simulink model "gm_uz_pmsm_model_9ph"  (R2021b)
settings: Solver=FixedStepAuto  StartTime=0.0  StopTime=0.8  RelTol=1e-3
PreLoadFcn:
  | uz_pmsm_model_9ph_init_parameter
undefined symbols (not defined in the file or in its folder): a, b, c, friction_coefficient, inertia, k_i_d, k_i_q, k_p_d, k_p_q, Kpd, L_d, L_o1, L_o2, L_q, L_x1, L_x2, L_y1, L_y2, L_zero, polepair, psi_pm, R_1, static_friction_torque, Tnd
libraries: hdlmdlgenlib x190, hdlsllib x90, dspsigops x17, simulink x3, slpidlib x2, spsAlphaBetaZerotodq0Lib x1, pid_lib x1, spsdq0toAlphaBetaZeroLib x1
(part 3 of 6)

== system gm_uz_pmsm_model_9ph/Subsystem8/Subsystem3 ==
  setp_Mod_x : Inport
  actual_Mod_x : Inport  Port=2
  Add : Sum  Inputs=+-
  Data Type Conversion8 : DataTypeConversion  OutDataTypeStr=double
  PID Controller2 : slpidlib/PID Controller  Controller=PI  Form=Ideal  TimeDomain=Continuous-time  UseExternalTs=off  SampleTime=-1  IntegratorMethod=Forward Euler  FilterMethod=Forward Euler  ControllerParametersSource=internal  P=k_p_q  I=k_i_q  D=0  UseFilter=on  N=100  TunerSelectOption=Transfer Function Based (PID Tuner App)  InitialConditionSource=internal  InitialConditionForIntegrator=0  InitialConditionForFilter=0  DifferentiatorICPrevScaledInput=0  ExternalReset=none  TrackingMode=off  Kt=1  LimitOutput=on  SatLimitsSource=internal  UpperSaturationLimit=100  LowerSaturationLimit=-100  LinearizeAsGain=on  AntiWindupMode=clamping  Kb=1  POutMin=[]  POutMax=[]  IOutMin=[]  IOutMax=[]  DOutMin=[]  DOutMax=[]  NOutMin=[]  NOutMax=[]  SumOutMin=[]  SumOutMax=[]  SaturationOutMin=[]  SaturationOutMax=[]  PParamMin=[]  PParamMax=[]  IParamMin=[]  IParamMax=[]  DParamMin=[]  DParamMax=[]  NParamMin=[]  NParamMax=[]  KbParamMin=[]  KbParamMax=[]  KtParamMin=[]  KtParamMax=[]  KbOutMin=[]  KbOutMax=[]  KtOutMin=[]  KtOutMax=[]  IntegratorOutMin=[]  IntegratorOutMax=[]  FilterOutMin=[]  FilterOutMax=[]  SumI1OutMin=[]  SumI1OutMax=[]  SumI2OutMin=[]  SumI2OutMax=[]  SumI3OutMin=[]  SumI3OutMax=[]  SumI4OutMin=[]  SumI4OutMax=[]  SumDOutMin=[]  SumDOutMax=[]  DifferentiatorOutMin=[]  DifferentiatorOutMax=[]  FilterDiffOutCoefMin=[]  FilterDiffOutCoefMax=[]  ReciprocalOutMin=[]  ReciprocalOutMax=[]  SumDenOutMin=[]  SumDenOutMax=[]  SumNumOutMin=[]  SumNumOutMax=[]  DivideOutMin=[]  DivideOutMax=[]  UdiffTsProdOutMin=[]  UdiffTsProdOutMax=[]  NTsProdOutMin=[]  NTsProdOutMax=[]  UintegralTsProdOutMin=[]  UintegralTsProdOutMax=[]  UngainTsProdOutMin=[]  UngainTsProdOutMax=[]  IntegratorContinuousStateAttributes=''  IntegratorStateMustResolveToSignalObject=off  IntegratorRTWStateStorageClass=Auto  FilterContinuousStateAttributes=''  FilterStateMustResolveToSignalObject=off  FilterRTWStateStorageClass=Auto  ParallelPVariant=Passthrough  IdealPVariant=InternalParameters  IVariant=InternalParameters  DVariant=Disabled  IntegratorVariant=Continuous  SatVariant=Enabled  AWVariant=ContClampingIdeal  PCopyVariant=InternalParamsIdeal  TRVariant=Disabled  FdbkBlocksVariant=Forward  IdealPFdbkVariant=Disabled  SatFdbkVariant=Disabled  DerivativeFilterVariant=Disabled  NVariant=Disabled  NCopyVariant=Disabled_SignalSpec  FilterICVariant=Disabled  IntegratorICVariant=InternalICs  ExternalResetVariant=Disabled  TRSumVariant=Passthrough  SumFdbkVariant=Disabled  SumVariant=Sum_PI  TsampFilterVariant=InternalTs  TsampNgainVariant=Passthrough  TsampIntegralVariant=Passthrough  ExternalSaturationOutDataTypeStr=Inherit: Same as second input
  out_mod_x : Outport
  wires:
  Add/1 -> Data Type Conversion8/1
  actual_Mod_x/1 -> Add/2
  Data Type Conversion8/1 -> PID Controller2/1
  setp_Mod_x/1 -> Add/1
  PID Controller2/1 -> out_mod_x/1

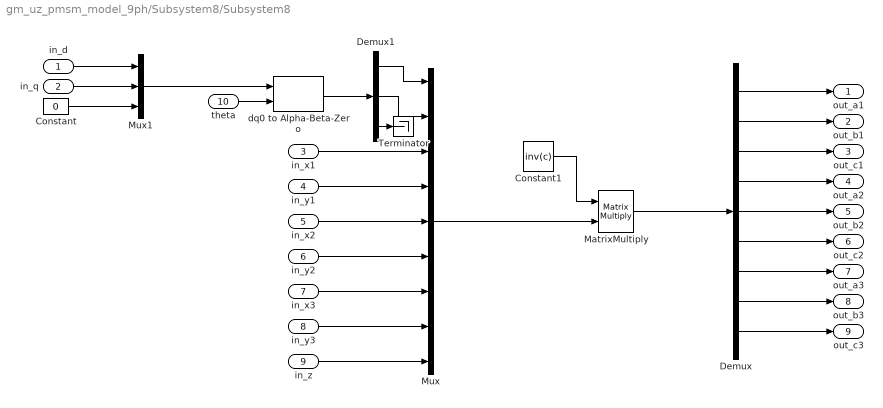
== system gm_uz_pmsm_model_9ph/Subsystem8/Subsystem8 ==
  in_d : Inport
  in_q : Inport  Port=2
  in_x1 : Inport  Port=3
  in_y1 : Inport  Port=4
  in_x2 : Inport  Port=5
  in_y2 : Inport  Port=6
  in_x3 : Inport  Port=7
  in_y3 : Inport  Port=8
  in_z : Inport  Port=9
  theta : Inport  Port=10
  Constant : Constant  Value=0
  Constant1 : Constant  Value=inv(c)
  Demux : Demux  Outputs=9
  Demux1 : Demux  Outputs=3
  MatrixMultiply : Product  Multiplication=Matrix(*)
  Mux : Mux  Inputs=9
  Mux1 : Mux  Inputs=3
  Terminator : Terminator
  dq0 to Alpha-Beta-Zero : spsdq0toAlphaBetaZeroLib/dq0 to Alpha-Beta-Zero  Alignment=90 degrees behind phase A axis
      settings: SourceProductBaseCode=PS
  out_a1 : Outport
  out_b1 : Outport  Port=2
  out_c1 : Outport  Port=3
  out_a2 : Outport  Port=4
  out_b2 : Outport  Port=5
  out_c2 : Outport  Port=6
  out_a3 : Outport  Port=7
  out_b3 : Outport  Port=8
  out_c3 : Outport  Port=9
  wires:
  Demux/7 -> out_a3/1
  Demux/9 -> out_c3/1
  Demux/8 -> out_b3/1
  Demux/5 -> out_b2/1
  Demux/6 -> out_c2/1
  Demux/4 -> out_a2/1
  Demux/3 -> out_c1/1
  Demux/2 -> out_b1/1
  Constant1/1 -> MatrixMultiply/1
  Demux1/3 -> Terminator/1
  Demux1/2 -> Mux/2
  Demux1/1 -> Mux/1
  dq0 to Alpha-Beta-Zero/1 -> Demux1/1
  theta/1 -> dq0 to Alpha-Beta-Zero/2
  Mux1/1 -> dq0 to Alpha-Beta-Zero/1
  in_d/1 -> Mux1/1
  in_q/1 -> Mux1/2
  Constant/1 -> Mux1/3
  in_z/1 -> Mux/9
  in_x2/1 -> Mux/5
  Mux/1 -> MatrixMultiply/2
  in_y1/1 -> Mux/4
  in_x1/1 -> Mux/3
  Demux/1 -> out_a1/1
  in_y2/1 -> Mux/6
  MatrixMultiply/1 -> Demux/1
  in_y3/1 -> Mux/8
  in_x3/1 -> Mux/7

== system gm_uz_pmsm_model_9ph/uz_pmsm_model_9ph/Add ==
  In1 : Inport
  In2 : Inport  Port=2
  Add : Sum  Inputs=+-  OutDataTypeStr=single  SampleTime=1e-08
  Add_pd1 : Delay  DelayLength=6
  Out1 : Outport
  wires:
  In1/1 -> Add/1
  In2/1 -> Add/2
  Add/1 -> Add_pd1/1
  Add_pd1/1 -> Out1/1

== system gm_uz_pmsm_model_9ph/uz_pmsm_model_9ph/Add1 ==
  In1 : Inport
  In2 : Inport  Port=2
  Add1 : Sum  Inputs=+-  OutDataTypeStr=single  SampleTime=1e-08
  Add1_pd1 : Delay  DelayLength=6
  Out1 : Outport
  wires:
  In1/1 -> Add1/1
  In2/1 -> Add1/2
  Add1/1 -> Add1_pd1/1
  Add1_pd1/1 -> Out1/1

== system gm_uz_pmsm_model_9ph/uz_pmsm_model_9ph/Add2 ==
  In1 : Inport
  In2 : Inport  Port=2
  Add2 : Sum  Inputs=+-  OutDataTypeStr=single  SampleTime=1e-08
  Add2_pd1 : Delay  DelayLength=6
  Out1 : Outport
  wires:
  In1/1 -> Add2/1
  In2/1 -> Add2/2
  Add2/1 -> Add2_pd1/1
  Add2_pd1/1 -> Out1/1

== system gm_uz_pmsm_model_9ph/uz_pmsm_model_9ph/Add3 ==
  In1 : Inport
  In2 : Inport  Port=2
  Add3 : Sum  Inputs=+-  OutDataTypeStr=single  SampleTime=1e-08
  Add3_pd1 : Delay  DelayLength=6
  Out1 : Outport
  wires:
  In1/1 -> Add3/1
  In2/1 -> Add3/2
  Add3/1 -> Add3_pd1/1
  Add3_pd1/1 -> Out1/1

== system gm_uz_pmsm_model_9ph/uz_pmsm_model_9ph/Add4 ==
  In1 : Inport
  In2 : Inport  Port=2
  Add4 : Sum  Inputs=+-  OutDataTypeStr=single  SampleTime=1e-08
  Add4_pd1 : Delay  DelayLength=6
  Out1 : Outport
  wires:
  In1/1 -> Add4/1
  In2/1 -> Add4/2
  Add4/1 -> Add4_pd1/1
  Add4_pd1/1 -> Out1/1

== system gm_uz_pmsm_model_9ph/uz_pmsm_model_9ph/Add5 ==
  In1 : Inport
  In2 : Inport  Port=2
  Add5 : Sum  Inputs=+-  OutDataTypeStr=single  SampleTime=1e-08
  Add5_pd1 : Delay  DelayLength=6
  Out1 : Outport
  wires:
  In1/1 -> Add5/1
  In2/1 -> Add5/2
  Add5/1 -> Add5_pd1/1
  Add5_pd1/1 -> Out1/1

== system gm_uz_pmsm_model_9ph/uz_pmsm_model_9ph/Add6 ==
  In1 : Inport
  In2 : Inport  Port=2
  Add6 : Sum  Inputs=+-  OutDataTypeStr=single  SampleTime=1e-08
  Add6_pd1 : Delay  DelayLength=6
  Out1 : Outport
  wires:
  In1/1 -> Add6/1
  In2/1 -> Add6/2
  Add6/1 -> Add6_pd1/1
  Add6_pd1/1 -> Out1/1

== system gm_uz_pmsm_model_9ph/uz_pmsm_model_9ph/Cast To Double ==
  In1 : Inport
  Cast To Double : DataTypeConversion  OutDataTypeStr=single  SampleTime=1e-08
  Cast To Double_pd1 : Delay  DelayLength=6
  Out1 : Outport
  wires:
  In1/1 -> Cast To Double/1
  Cast To Double/1 -> Cast To Double_pd1/1
  Cast To Double_pd1/1 -> Out1/1

== system gm_uz_pmsm_model_9ph/uz_pmsm_model_9ph/Cast To Double1 ==
  In1 : Inport
  Cast To Double1 : DataTypeConversion  OutDataTypeStr=single  SampleTime=1e-08
  Cast To Double1_pd1 : Delay  DelayLength=6
  Out1 : Outport
  wires:
  In1/1 -> Cast To Double1/1
  Cast To Double1/1 -> Cast To Double1_pd1/1
  Cast To Double1_pd1/1 -> Out1/1

== system gm_uz_pmsm_model_9ph/uz_pmsm_model_9ph/Cast To Double2 ==
  In1 : Inport
  Cast To Double2 : DataTypeConversion  OutDataTypeStr=single  SampleTime=1e-08
  Cast To Double2_pd1 : Delay  DelayLength=6
  Out1 : Outport
  wires:
  In1/1 -> Cast To Double2/1
  Cast To Double2/1 -> Cast To Double2_pd1/1
  Cast To Double2_pd1/1 -> Out1/1

== system gm_uz_pmsm_model_9ph/uz_pmsm_model_9ph/Data Type Conversion1 ==
  In1 : Inport
  Data Type Conversion1 : DataTypeConversion  OutDataTypeStr=fixdt(1, 25, 12)  RndMeth=Nearest  SampleTime=1e-08
  Data Type Conversion1_pd1 : Delay  DelayLength=6
  Out1 : Outport
  wires:
  In1/1 -> Data Type Conversion1/1
  Data Type Conversion1/1 -> Data Type Conversion1_pd1/1
  Data Type Conversion1_pd1/1 -> Out1/1

== system gm_uz_pmsm_model_9ph/uz_pmsm_model_9ph/Data Type Conversion11 ==
  In1 : Inport
  Data Type Conversion11 : DataTypeConversion  OutDataTypeStr=double  RndMeth=Nearest  SampleTime=1e-08
  Data Type Conversion11_pd1 : Delay  DelayLength=3
  Out1 : Outport
  wires:
  In1/1 -> Data Type Conversion11/1
  Data Type Conversion11/1 -> Data Type Conversion11_pd1/1
  Data Type Conversion11_pd1/1 -> Out1/1

== system gm_uz_pmsm_model_9ph/uz_pmsm_model_9ph/Data Type Conversion12 ==
  In1 : Inport
  Data Type Conversion12 : DataTypeConversion  OutDataTypeStr=double  RndMeth=Nearest  SampleTime=1e-08
  Data Type Conversion12_pd1 : Delay  DelayLength=3
  Out1 : Outport
  wires:
  In1/1 -> Data Type Conversion12/1
  Data Type Conversion12/1 -> Data Type Conversion12_pd1/1
  Data Type Conversion12_pd1/1 -> Out1/1

== system gm_uz_pmsm_model_9ph/uz_pmsm_model_9ph/Data Type Conversion13 ==
  In1 : Inport
  Data Type Conversion13 : DataTypeConversion  OutDataTypeStr=single  RndMeth=Nearest  SampleTime=1e-08
  Data Type Conversion13_pd1 : Delay  DelayLength=3
  Out1 : Outport
  wires:
  In1/1 -> Data Type Conversion13/1
  Data Type Conversion13/1 -> Data Type Conversion13_pd1/1
  Data Type Conversion13_pd1/1 -> Out1/1

== system gm_uz_pmsm_model_9ph/uz_pmsm_model_9ph/Data Type Conversion14 ==
  In1 : Inport
  Data Type Conversion14 : DataTypeConversion  OutDataTypeStr=double  RndMeth=Nearest  SampleTime=1e-08
  Data Type Conversion14_pd1 : Delay  DelayLength=3
  Out1 : Outport
  wires:
  In1/1 -> Data Type Conversion14/1
  Data Type Conversion14/1 -> Data Type Conversion14_pd1/1
  Data Type Conversion14_pd1/1 -> Out1/1

== system gm_uz_pmsm_model_9ph/uz_pmsm_model_9ph/Data Type Conversion141 ==
  In1 : Inport
  Data Type Conversion141 : DataTypeConversion  OutDataTypeStr=single  RndMeth=Nearest  SampleTime=1e-08
  Data Type Conversion141_pd1 : Delay  DelayLength=3
  Out1 : Outport
  wires:
  In1/1 -> Data Type Conversion141/1
  Data Type Conversion141/1 -> Data Type Conversion141_pd1/1
  Data Type Conversion141_pd1/1 -> Out1/1

== system gm_uz_pmsm_model_9ph/uz_pmsm_model_9ph/Data Type Conversion15 ==
  In1 : Inport
  Data Type Conversion15 : DataTypeConversion  OutDataTypeStr=single  RndMeth=Nearest  SampleTime=1e-08
  Data Type Conversion15_pd1 : Delay  DelayLength=3
  Out1 : Outport
  wires:
  In1/1 -> Data Type Conversion15/1
  Data Type Conversion15/1 -> Data Type Conversion15_pd1/1
  Data Type Conversion15_pd1/1 -> Out1/1

== system gm_uz_pmsm_model_9ph/uz_pmsm_model_9ph/Data Type Conversion16 ==
  In1 : Inport
  Data Type Conversion16 : DataTypeConversion  OutDataTypeStr=single  RndMeth=Nearest  SampleTime=1e-08
  Data Type Conversion16_pd1 : Delay  DelayLength=3
  Out1 : Outport
  wires:
  In1/1 -> Data Type Conversion16/1
  Data Type Conversion16/1 -> Data Type Conversion16_pd1/1
  Data Type Conversion16_pd1/1 -> Out1/1

== system gm_uz_pmsm_model_9ph/uz_pmsm_model_9ph/Data Type Conversion17 ==
  In1 : Inport
  Data Type Conversion17 : DataTypeConversion  OutDataTypeStr=single  RndMeth=Nearest  SampleTime=1e-08
  Data Type Conversion17_pd1 : Delay  DelayLength=3
  Out1 : Outport
  wires:
  In1/1 -> Data Type Conversion17/1
  Data Type Conversion17/1 -> Data Type Conversion17_pd1/1
  Data Type Conversion17_pd1/1 -> Out1/1

== system gm_uz_pmsm_model_9ph/uz_pmsm_model_9ph/Data Type Conversion18 ==
  In1 : Inport
  Data Type Conversion18 : DataTypeConversion  OutDataTypeStr=single  RndMeth=Nearest  SampleTime=1e-08
  Data Type Conversion18_pd1 : Delay  DelayLength=3
  Out1 : Outport
  wires:
  In1/1 -> Data Type Conversion18/1
  Data Type Conversion18/1 -> Data Type Conversion18_pd1/1
  Data Type Conversion18_pd1/1 -> Out1/1

== system gm_uz_pmsm_model_9ph/uz_pmsm_model_9ph/Data Type Conversion19 ==
  In1 : Inport
  Data Type Conversion19 : DataTypeConversion  OutDataTypeStr=single  RndMeth=Nearest  SampleTime=1e-08
  Data Type Conversion19_pd1 : Delay  DelayLength=3
  Out1 : Outport
  wires:
  In1/1 -> Data Type Conversion19/1
  Data Type Conversion19/1 -> Data Type Conversion19_pd1/1
  Data Type Conversion19_pd1/1 -> Out1/1

== system gm_uz_pmsm_model_9ph/uz_pmsm_model_9ph/Data Type Conversion20 ==
  In1 : Inport
  Data Type Conversion20 : DataTypeConversion  OutDataTypeStr=single  RndMeth=Nearest  SampleTime=1e-08
  Data Type Conversion20_pd1 : Delay  DelayLength=3
  Out1 : Outport
  wires:
  In1/1 -> Data Type Conversion20/1
  Data Type Conversion20/1 -> Data Type Conversion20_pd1/1
  Data Type Conversion20_pd1/1 -> Out1/1

== system gm_uz_pmsm_model_9ph/uz_pmsm_model_9ph/Data Type Conversion21 ==
  In1 : Inport
  Data Type Conversion21 : DataTypeConversion  OutDataTypeStr=double  RndMeth=Nearest  SampleTime=1e-08
  Data Type Conversion21_pd1 : Delay  DelayLength=3
  Out1 : Outport
  wires:
  In1/1 -> Data Type Conversion21/1
  Data Type Conversion21/1 -> Data Type Conversion21_pd1/1
  Data Type Conversion21_pd1/1 -> Out1/1

== system gm_uz_pmsm_model_9ph/uz_pmsm_model_9ph/Data Type Conversion22 ==
  In1 : Inport
  Data Type Conversion22 : DataTypeConversion  OutDataTypeStr=double  RndMeth=Nearest  SampleTime=1e-08
  Data Type Conversion22_pd1 : Delay  DelayLength=3
  Out1 : Outport
  wires:
  In1/1 -> Data Type Conversion22/1
  Data Type Conversion22/1 -> Data Type Conversion22_pd1/1
  Data Type Conversion22_pd1/1 -> Out1/1

== system gm_uz_pmsm_model_9ph/uz_pmsm_model_9ph/Data Type Conversion23 ==
  In1 : Inport
  Data Type Conversion23 : DataTypeConversion  OutDataTypeStr=single  RndMeth=Nearest  SampleTime=1e-08
  Data Type Conversion23_pd1 : Delay  DelayLength=3
  Out1 : Outport
  wires:
  In1/1 -> Data Type Conversion23/1
  Data Type Conversion23/1 -> Data Type Conversion23_pd1/1
  Data Type Conversion23_pd1/1 -> Out1/1

== system gm_uz_pmsm_model_9ph/uz_pmsm_model_9ph/Data Type Conversion24 ==
  In1 : Inport
  Data Type Conversion24 : DataTypeConversion  OutDataTypeStr=double  RndMeth=Nearest  SampleTime=1e-08
  Data Type Conversion24_pd1 : Delay  DelayLength=3
  Out1 : Outport
  wires:
  In1/1 -> Data Type Conversion24/1
  Data Type Conversion24/1 -> Data Type Conversion24_pd1/1
  Data Type Conversion24_pd1/1 -> Out1/1

== system gm_uz_pmsm_model_9ph/uz_pmsm_model_9ph/Data Type Conversion25 ==
  In1 : Inport
  Data Type Conversion25 : DataTypeConversion  OutDataTypeStr=double  RndMeth=Nearest  SampleTime=1e-08
  Data Type Conversion25_pd1 : Delay  DelayLength=3
  Out1 : Outport
  wires:
  In1/1 -> Data Type Conversion25/1
  Data Type Conversion25/1 -> Data Type Conversion25_pd1/1
  Data Type Conversion25_pd1/1 -> Out1/1

== system gm_uz_pmsm_model_9ph/uz_pmsm_model_9ph/Data Type Conversion26 ==
  In1 : Inport
  Data Type Conversion26 : DataTypeConversion  OutDataTypeStr=double  RndMeth=Nearest  SampleTime=1e-08
  Data Type Conversion26_pd1 : Delay  DelayLength=3
  Out1 : Outport
  wires:
  In1/1 -> Data Type Conversion26/1
  Data Type Conversion26/1 -> Data Type Conversion26_pd1/1
  Data Type Conversion26_pd1/1 -> Out1/1

== system gm_uz_pmsm_model_9ph/uz_pmsm_model_9ph/Data Type Conversion27 ==
  In1 : Inport
  Data Type Conversion27 : DataTypeConversion  OutDataTypeStr=double  RndMeth=Nearest  SampleTime=1e-08
  Data Type Conversion27_pd1 : Delay  DelayLength=3
  Out1 : Outport
  wires:
  In1/1 -> Data Type Conversion27/1
  Data Type Conversion27/1 -> Data Type Conversion27_pd1/1
  Data Type Conversion27_pd1/1 -> Out1/1

== system gm_uz_pmsm_model_9ph/uz_pmsm_model_9ph/Data Type Conversion28 ==
  In1 : Inport
  Data Type Conversion28 : DataTypeConversion  OutDataTypeStr=double  RndMeth=Nearest  SampleTime=1e-08
  Data Type Conversion28_pd1 : Delay  DelayLength=3
  Out1 : Outport
  wires:
  In1/1 -> Data Type Conversion28/1
  Data Type Conversion28/1 -> Data Type Conversion28_pd1/1
  Data Type Conversion28_pd1/1 -> Out1/1

== system gm_uz_pmsm_model_9ph/uz_pmsm_model_9ph/Data Type Conversion29 ==
  In1 : Inport
  Data Type Conversion29 : DataTypeConversion  OutDataTypeStr=double  RndMeth=Nearest  SampleTime=1e-08
  Data Type Conversion29_pd1 : Delay  DelayLength=3
  Out1 : Outport
  wires:
  In1/1 -> Data Type Conversion29/1
  Data Type Conversion29/1 -> Data Type Conversion29_pd1/1
  Data Type Conversion29_pd1/1 -> Out1/1

== system gm_uz_pmsm_model_9ph/uz_pmsm_model_9ph/Data Type Conversion3 ==
  In1 : Inport
  Data Type Conversion3 : DataTypeConversion  OutDataTypeStr=double  RndMeth=Nearest  SampleTime=1e-08
  Data Type Conversion3_pd1 : Delay  DelayLength=3
  Out1 : Outport
  wires:
  In1/1 -> Data Type Conversion3/1
  Data Type Conversion3/1 -> Data Type Conversion3_pd1/1
  Data Type Conversion3_pd1/1 -> Out1/1

== system gm_uz_pmsm_model_9ph/uz_pmsm_model_9ph/Data Type Conversion30 ==
  In1 : Inport
  Data Type Conversion30 : DataTypeConversion  OutDataTypeStr=double  RndMeth=Nearest  SampleTime=1e-08
  Data Type Conversion30_pd1 : Delay  DelayLength=3
  Out1 : Outport
  wires:
  In1/1 -> Data Type Conversion30/1
  Data Type Conversion30/1 -> Data Type Conversion30_pd1/1
  Data Type Conversion30_pd1/1 -> Out1/1

== system gm_uz_pmsm_model_9ph/uz_pmsm_model_9ph/Data Type Conversion31 ==
  In1 : Inport
  Data Type Conversion31 : DataTypeConversion  OutDataTypeStr=single  RndMeth=Nearest  SampleTime=1e-08
  Data Type Conversion31_pd1 : Delay  DelayLength=3
  Out1 : Outport
  wires:
  In1/1 -> Data Type Conversion31/1
  Data Type Conversion31/1 -> Data Type Conversion31_pd1/1
  Data Type Conversion31_pd1/1 -> Out1/1

== system gm_uz_pmsm_model_9ph/uz_pmsm_model_9ph/Data Type Conversion32 ==
  In1 : Inport
  Data Type Conversion32 : DataTypeConversion  OutDataTypeStr=single  RndMeth=Nearest  SampleTime=1e-08
  Data Type Conversion32_pd1 : Delay  DelayLength=3
  Out1 : Outport
  wires:
  In1/1 -> Data Type Conversion32/1
  Data Type Conversion32/1 -> Data Type Conversion32_pd1/1
  Data Type Conversion32_pd1/1 -> Out1/1

== system gm_uz_pmsm_model_9ph/uz_pmsm_model_9ph/Data Type Conversion33 ==
  In1 : Inport
  Data Type Conversion33 : DataTypeConversion  OutDataTypeStr=double  RndMeth=Nearest  SampleTime=1e-08
  Data Type Conversion33_pd1 : Delay  DelayLength=3
  Out1 : Outport
  wires:
  In1/1 -> Data Type Conversion33/1
  Data Type Conversion33/1 -> Data Type Conversion33_pd1/1
  Data Type Conversion33_pd1/1 -> Out1/1

== system gm_uz_pmsm_model_9ph/uz_pmsm_model_9ph/Data Type Conversion331 ==
  In1 : Inport
  Data Type Conversion331 : DataTypeConversion  OutDataTypeStr=double  RndMeth=Nearest  SampleTime=1e-08
  Data Type Conversion331_pd1 : Delay  DelayLength=3
  Out1 : Outport
  wires:
  In1/1 -> Data Type Conversion331/1
  Data Type Conversion331/1 -> Data Type Conversion331_pd1/1
  Data Type Conversion331_pd1/1 -> Out1/1

== system gm_uz_pmsm_model_9ph/uz_pmsm_model_9ph/Data Type Conversion37 ==
  In1 : Inport
  Data Type Conversion37 : DataTypeConversion  OutDataTypeStr=single  RndMeth=Nearest  SampleTime=1e-08
  Data Type Conversion37_pd1 : Delay  DelayLength=6
  Out1 : Outport
  wires:
  In1/1 -> Data Type Conversion37/1
  Data Type Conversion37/1 -> Data Type Conversion37_pd1/1
  Data Type Conversion37_pd1/1 -> Out1/1

== system gm_uz_pmsm_model_9ph/uz_pmsm_model_9ph/Data Type Conversion5 ==
  In1 : Inport
  Data Type Conversion5 : DataTypeConversion  OutDataTypeStr=double  RndMeth=Nearest  SampleTime=1e-08
  Data Type Conversion5_pd1 : Delay  DelayLength=3
  Out1 : Outport
  wires:
  In1/1 -> Data Type Conversion5/1
  Data Type Conversion5/1 -> Data Type Conversion5_pd1/1
  Data Type Conversion5_pd1/1 -> Out1/1

== system gm_uz_pmsm_model_9ph/uz_pmsm_model_9ph/Data Type Conversion8 ==
  In1 : Inport
  Data Type Conversion8 : DataTypeConversion  OutDataTypeStr=single  RndMeth=Nearest  SampleTime=1e-08
  Data Type Conversion8_pd1 : Delay  DelayLength=3
  Out1 : Outport
  wires:
  In1/1 -> Data Type Conversion8/1
  Data Type Conversion8/1 -> Data Type Conversion8_pd1/1
  Data Type Conversion8_pd1/1 -> Out1/1

== system gm_uz_pmsm_model_9ph/uz_pmsm_model_9ph/Data Type Conversion9 ==
  In1 : Inport
  Data Type Conversion9 : DataTypeConversion  OutDataTypeStr=fixdt(1, 25, 12)  RndMeth=Nearest  SampleTime=1e-08
  Data Type Conversion9_pd1 : Delay  DelayLength=6
  Out1 : Outport
  wires:
  In1/1 -> Data Type Conversion9/1
  Data Type Conversion9/1 -> Data Type Conversion9_pd1/1
  Data Type Conversion9_pd1/1 -> Out1/1

== system gm_uz_pmsm_model_9ph/uz_pmsm_model_9ph/Divide ==
  In1 : Inport
  In2 : Inport  Port=2
  Divide : Product  Inputs=**  OutDataTypeStr=single  SampleTime=1e-08
  Divide_pd1 : Delay  DelayLength=6
  Out1 : Outport
  wires:
  In1/1 -> Divide/1
  In2/1 -> Divide/2
  Divide/1 -> Divide_pd1/1
  Divide_pd1/1 -> Out1/1

== system gm_uz_pmsm_model_9ph/uz_pmsm_model_9ph/Divide1 ==
  In1 : Inport
  In2 : Inport  Port=2
  Divide1 : Product  Inputs=**  OutDataTypeStr=single  SampleTime=1e-08
  Divide1_pd1 : Delay  DelayLength=6
  Out1 : Outport
  wires:
  In1/1 -> Divide1/1
  In2/1 -> Divide1/2
  Divide1/1 -> Divide1_pd1/1
  Divide1_pd1/1 -> Out1/1

== system gm_uz_pmsm_model_9ph/uz_pmsm_model_9ph/Divide10 ==
  In1 : Inport
  In2 : Inport  Port=2
  Divide10 : Product  Inputs=**  OutDataTypeStr=single  SampleTime=1e-08
  Divide10_pd1 : Delay  DelayLength=6
  Out1 : Outport
  wires:
  In1/1 -> Divide10/1
  In2/1 -> Divide10/2
  Divide10/1 -> Divide10_pd1/1
  Divide10_pd1/1 -> Out1/1

== system gm_uz_pmsm_model_9ph/uz_pmsm_model_9ph/Divide11 ==
  In1 : Inport
  In2 : Inport  Port=2
  Divide11 : Product  Inputs=**  OutDataTypeStr=single  SampleTime=1e-08
  Divide11_pd1 : Delay  DelayLength=6
  Out1 : Outport
  wires:
  In1/1 -> Divide11/1
  In2/1 -> Divide11/2
  Divide11/1 -> Divide11_pd1/1
  Divide11_pd1/1 -> Out1/1

== system gm_uz_pmsm_model_9ph/uz_pmsm_model_9ph/Divide12 ==
  In1 : Inport
  In2 : Inport  Port=2
  Divide12 : Product  Inputs=**  OutDataTypeStr=single  SampleTime=1e-08
  Divide12_pd1 : Delay  DelayLength=6
  Out1 : Outport
  wires:
  In1/1 -> Divide12/1
  In2/1 -> Divide12/2
  Divide12/1 -> Divide12_pd1/1
  Divide12_pd1/1 -> Out1/1

== system gm_uz_pmsm_model_9ph/uz_pmsm_model_9ph/Divide13 ==
  In1 : Inport
  In2 : Inport  Port=2
  Divide13 : Product  Inputs=**  OutDataTypeStr=single  SampleTime=1e-08
  Divide13_pd1 : Delay  DelayLength=6
  Out1 : Outport
  wires:
  In1/1 -> Divide13/1
  In2/1 -> Divide13/2
  Divide13/1 -> Divide13_pd1/1
  Divide13_pd1/1 -> Out1/1

== system gm_uz_pmsm_model_9ph/uz_pmsm_model_9ph/Divide2 ==
  In1 : Inport
  In2 : Inport  Port=2
  Divide2 : Product  Inputs=**  OutDataTypeStr=single  SampleTime=1e-08
  Divide2_pd1 : Delay  DelayLength=6
  Out1 : Outport
  wires:
  In1/1 -> Divide2/1
  In2/1 -> Divide2/2
  Divide2/1 -> Divide2_pd1/1
  Divide2_pd1/1 -> Out1/1

== system gm_uz_pmsm_model_9ph/uz_pmsm_model_9ph/Divide3 ==
  In1 : Inport
  In2 : Inport  Port=2
  Divide3 : Product  Inputs=**  OutDataTypeStr=single  SampleTime=1e-08
  Divide3_pd1 : Delay  DelayLength=6
  Out1 : Outport
  wires:
  In1/1 -> Divide3/1
  In2/1 -> Divide3/2
  Divide3/1 -> Divide3_pd1/1
  Divide3_pd1/1 -> Out1/1

== system gm_uz_pmsm_model_9ph/uz_pmsm_model_9ph/Divide4 ==
  In1 : Inport
  In2 : Inport  Port=2
  Divide4 : Product  Inputs=**  OutDataTypeStr=single  SampleTime=1e-08
  Divide4_pd1 : Delay  DelayLength=6
  Out1 : Outport
  wires:
  In1/1 -> Divide4/1
  In2/1 -> Divide4/2
  Divide4/1 -> Divide4_pd1/1
  Divide4_pd1/1 -> Out1/1

== system gm_uz_pmsm_model_9ph/uz_pmsm_model_9ph/Divide5 ==
  In1 : Inport
  In2 : Inport  Port=2
  Divide5 : Product  Inputs=**  OutDataTypeStr=single  SampleTime=1e-08
  Divide5_pd1 : Delay  DelayLength=6
  Out1 : Outport
  wires:
  In1/1 -> Divide5/1
  In2/1 -> Divide5/2
  Divide5/1 -> Divide5_pd1/1
  Divide5_pd1/1 -> Out1/1

== system gm_uz_pmsm_model_9ph/uz_pmsm_model_9ph/Divide6 ==
  In1 : Inport
  In2 : Inport  Port=2
  Divide6 : Product  Inputs=**  OutDataTypeStr=single  SampleTime=1e-08
  Divide6_pd1 : Delay  DelayLength=6
  Out1 : Outport
  wires:
  In1/1 -> Divide6/1
  In2/1 -> Divide6/2
  Divide6/1 -> Divide6_pd1/1
  Divide6_pd1/1 -> Out1/1

== system gm_uz_pmsm_model_9ph/uz_pmsm_model_9ph/Divide7 ==
  In1 : Inport
  In2 : Inport  Port=2
  Divide7 : Product  Inputs=**  OutDataTypeStr=single  SampleTime=1e-08
  Divide7_pd1 : Delay  DelayLength=6
  Out1 : Outport
  wires:
  In1/1 -> Divide7/1
  In2/1 -> Divide7/2
  Divide7/1 -> Divide7_pd1/1
  Divide7_pd1/1 -> Out1/1

== system gm_uz_pmsm_model_9ph/uz_pmsm_model_9ph/Divide8 ==
  In1 : Inport
  In2 : Inport  Port=2
  Divide8 : Product  Inputs=**  OutDataTypeStr=single  SampleTime=1e-08
  Divide8_pd1 : Delay  DelayLength=6
  Out1 : Outport
  wires:
  In1/1 -> Divide8/1
  In2/1 -> Divide8/2
  Divide8/1 -> Divide8_pd1/1
  Divide8_pd1/1 -> Out1/1

== system gm_uz_pmsm_model_9ph/uz_pmsm_model_9ph/Divide9 ==
  In1 : Inport
  In2 : Inport  Port=2
  Divide9 : Product  Inputs=**  OutDataTypeStr=single  SampleTime=1e-08
  Divide9_pd1 : Delay  DelayLength=6
  Out1 : Outport
  wires:
  In1/1 -> Divide9/1
  In2/1 -> Divide9/2
  Divide9/1 -> Divide9_pd1/1
  Divide9_pd1/1 -> Out1/1

== system gm_uz_pmsm_model_9ph/uz_pmsm_model_9ph/Factor ==
  In1 : Inport
  In2 : Inport  Port=2
  Factor : Product  Inputs=**  OutDataTypeStr=single  SampleTime=1e-08
  Factor_pd1 : Delay  DelayLength=6
  Out1 : Outport
  wires:
  In1/1 -> Factor/1
  In2/1 -> Factor/2
  Factor/1 -> Factor_pd1/1
  Factor_pd1/1 -> Out1/1

== system gm_uz_pmsm_model_9ph/uz_pmsm_model_9ph/Gain ==
  In1 : Inport
  In2 : Inport  Port=2
  Gain : Product  Inputs=**  OutDataTypeStr=double  SampleTime=1e-08
  Gain_pd1 : Delay  DelayLength=6
  Out1 : Outport
  wires:
  In1/1 -> Gain/1
  In2/1 -> Gain/2
  Gain/1 -> Gain_pd1/1
  Gain_pd1/1 -> Out1/1

== system gm_uz_pmsm_model_9ph/uz_pmsm_model_9ph/Gain1 ==
  In1 : Inport
  In2 : Inport  Port=2
  Gain1 : Product  Inputs=**  OutDataTypeStr=double  SampleTime=1e-08
  Gain1_pd1 : Delay  DelayLength=6
  Out1 : Outport
  wires:
  In1/1 -> Gain1/1
  In2/1 -> Gain1/2
  Gain1/1 -> Gain1_pd1/1
  Gain1_pd1/1 -> Out1/1

== system gm_uz_pmsm_model_9ph/uz_pmsm_model_9ph/Gain2 ==
  In1 : Inport
  In2 : Inport  Port=2
  Gain2 : Product  Inputs=**  OutDataTypeStr=double  SampleTime=1e-08
  Gain2_pd1 : Delay  DelayLength=6
  Out1 : Outport
  wires:
  In1/1 -> Gain2/1
  In2/1 -> Gain2/2
  Gain2/1 -> Gain2_pd1/1
  Gain2_pd1/1 -> Out1/1

== system gm_uz_pmsm_model_9ph/uz_pmsm_model_9ph/Gain3 ==
  In1 : Inport
  In2 : Inport  Port=2
  Gain3 : Product  Inputs=**  OutDataTypeStr=double  SampleTime=1e-08
  Gain3_pd1 : Delay  DelayLength=6
  Out1 : Outport
  wires:
  In1/1 -> Gain3/1
  In2/1 -> Gain3/2
  Gain3/1 -> Gain3_pd1/1
  Gain3_pd1/1 -> Out1/1

== system gm_uz_pmsm_model_9ph/uz_pmsm_model_9ph/Gain4 ==
  In1 : Inport
  In2 : Inport  Port=2
  Gain4 : Product  Inputs=**  OutDataTypeStr=double  SampleTime=1e-08
  Gain4_pd1 : Delay  DelayLength=6
  Out1 : Outport
  wires:
  In1/1 -> Gain4/1
  In2/1 -> Gain4/2
  Gain4/1 -> Gain4_pd1/1
  Gain4_pd1/1 -> Out1/1

== system gm_uz_pmsm_model_9ph/uz_pmsm_model_9ph/Gain5 ==
  In1 : Inport
  In2 : Inport  Port=2
  Gain5 : Product  Inputs=**  OutDataTypeStr=double  SampleTime=1e-08
  Gain5_pd1 : Delay  DelayLength=6
  Out1 : Outport
  wires:
  In1/1 -> Gain5/1
  In2/1 -> Gain5/2
  Gain5/1 -> Gain5_pd1/1
  Gain5_pd1/1 -> Out1/1

== system gm_uz_pmsm_model_9ph/uz_pmsm_model_9ph/Gain6 ==
  In1 : Inport
  In2 : Inport  Port=2
  Gain6 : Product  Inputs=**  OutDataTypeStr=double  SampleTime=1e-08
  Gain6_pd1 : Delay  DelayLength=6
  Out1 : Outport
  wires:
  In1/1 -> Gain6/1
  In2/1 -> Gain6/2
  Gain6/1 -> Gain6_pd1/1
  Gain6_pd1/1 -> Out1/1

== system gm_uz_pmsm_model_9ph/uz_pmsm_model_9ph/Gain7 ==
  In1 : Inport
  In2 : Inport  Port=2
  Gain7 : Product  Inputs=**  OutDataTypeStr=double  SampleTime=1e-08
  Gain7_pd1 : Delay  DelayLength=6
  Out1 : Outport
  wires:
  In1/1 -> Gain7/1
  In2/1 -> Gain7/2
  Gain7/1 -> Gain7_pd1/1
  Gain7_pd1/1 -> Out1/1

== system gm_uz_pmsm_model_9ph/uz_pmsm_model_9ph/Gain8 ==
  In1 : Inport
  In2 : Inport  Port=2
  Gain8 : Product  Inputs=**  OutDataTypeStr=double  SampleTime=1e-08
  Gain8_pd1 : Delay  DelayLength=6
  Out1 : Outport
  wires:
  In1/1 -> Gain8/1
  In2/1 -> Gain8/2
  Gain8/1 -> Gain8_pd1/1
  Gain8_pd1/1 -> Out1/1

== system gm_uz_pmsm_model_9ph/uz_pmsm_model_9ph/Gain9 ==
  In1 : Inport
  In2 : Inport  Port=2
  Gain9 : Product  Inputs=**  OutDataTypeStr=double  SampleTime=1e-08
  Gain9_pd1 : Delay  DelayLength=6
  Out1 : Outport
  wires:
  In1/1 -> Gain9/1
  In2/1 -> Gain9/2
  Gain9/1 -> Gain9_pd1/1
  Gain9_pd1/1 -> Out1/1

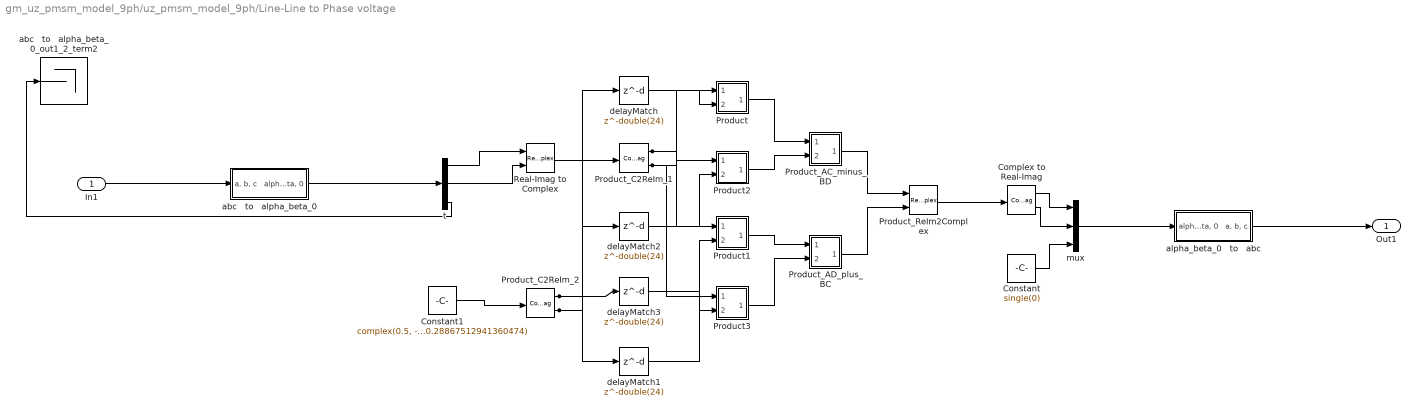
== system gm_uz_pmsm_model_9ph/uz_pmsm_model_9ph/Line-Line to Phase voltage ==
  In1 : Inport  OutDataTypeStr=single  PortDimensions=[3]  SampleTime=1e-08
  Complex to Real-Imag : ComplexToRealImag  SampleTime=1e-08
  Constant : Constant  Value=single(0)  OutDataTypeStr=single  SampleTime=1e-08
  Constant1 : Constant  Value=complex(0.5, -0.28867512941360474)  OutDataTypeStr=single  SampleTime=1e-08
  Product : Subsystem
      mask Display: disp('NFP\nmul');
  Product1 : Subsystem
      mask Display: disp('NFP\nmul');
  Product2 : Subsystem
      mask Display: disp('NFP\nmul');
  Product3 : Subsystem
      mask Display: disp('NFP\nmul');
  Product_AC_minus_BD : Subsystem
      mask Display: disp('NFP\nadd');
  Product_AD_plus_BC : Subsystem
      mask Display: disp('NFP\nadd');
  Product_C2ReIm_1 : ComplexToRealImag  SampleTime=1e-08
  Product_C2ReIm_2 : ComplexToRealImag  SampleTime=1e-08
  Product_ReIm2Complex : RealImagToComplex  SampleTime=1e-08
  Real-Imag to Complex : RealImagToComplex  ConstantPart=single(0)  SampleTime=1e-08
  abc   to   alpha_beta_0 : Subsystem
  abc   to   alpha_beta_0_out1_2_term2 : Terminator
  alpha_beta_0   to   abc : Subsystem
  delayMatch{,1..3} (4 alike) : Delay  DelayLength=double(24)  InitialCondition=0  SampleTime=1e-08
  mux : Mux  Inputs=3
  t : Demux  Outputs=3
  Out1 : Outport  SampleTime=1e-08
  wires:
  Complex to Real-Imag/1 -> mux/1
  Complex to Real-Imag/2 -> mux/2
  Constant/1 -> mux/3
  Constant1/1 -> Product_C2ReIm_2/1
  mux/1 -> alpha_beta_0   to   abc/1("alpha, beta, 0  ")
  Product_ReIm2Complex/1 -> Complex to Real-Imag/1
  Real-Imag to Complex/1 -> Product_C2ReIm_1/1
  abc   to   alpha_beta_0/1("alpha, beta, 0 ") -> t/1
  alpha_beta_0   to   abc/1("a, b, c") -> Out1/1
  t/1 -> Real-Imag to Complex/1
  t/2 -> Real-Imag to Complex/2
  t/3 -> abc   to   alpha_beta_0_out1_2_term2/1
  Product_C2ReIm_1/1 -> Product1/1(In1), Product/1(In1)
  Product_C2ReIm_1/2 -> Product3/1(In1), Product2/1(In1)
  delayMatch/1 -> Product/2(In2)
  delayMatch1/1 -> Product1/2(In2)
  delayMatch3/1 -> Product3/2(In2)
  delayMatch2/1 -> Product2/2(In2)
  Product_C2ReIm_2/2 -> delayMatch2/1, delayMatch1/1
  Product_C2ReIm_2/1 -> delayMatch3/1, delayMatch/1
  Product/1(Out1) -> Product_AC_minus_BD/1(In1)
  Product1/1(Out1) -> Product_AD_plus_BC/1(In1)
  Product2/1(Out1) -> Product_AC_minus_BD/2(In2)
  Product3/1(Out1) -> Product_AD_plus_BC/2(In2)
  Product_AC_minus_BD/1(Out1) -> Product_ReIm2Complex/1
  Product_AD_plus_BC/1(Out1) -> Product_ReIm2Complex/2
  In1/1 -> abc   to   alpha_beta_0/1("a, b, c")

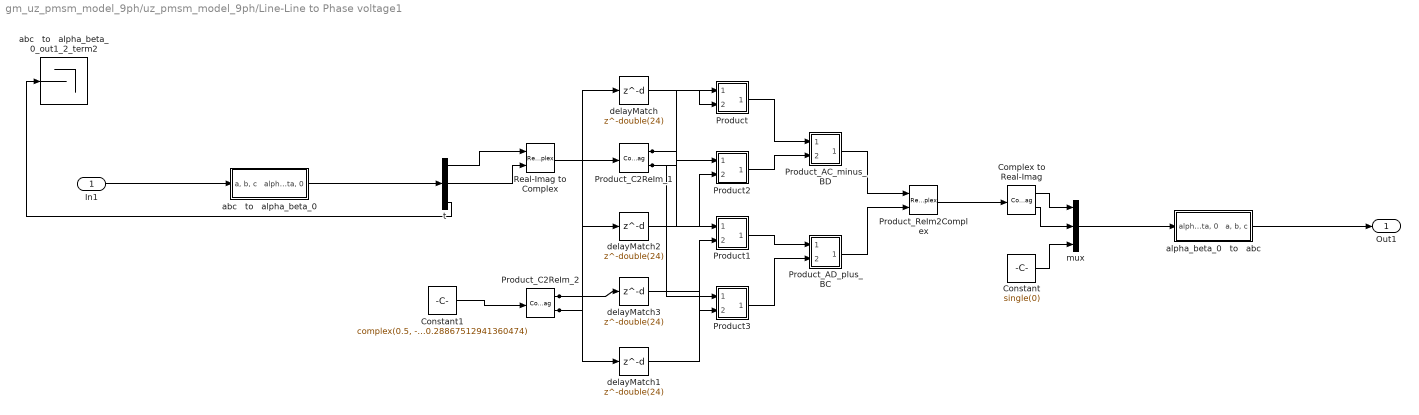
== system gm_uz_pmsm_model_9ph/uz_pmsm_model_9ph/Line-Line to Phase voltage1 ==
  In1 : Inport  OutDataTypeStr=single  PortDimensions=[3]  SampleTime=1e-08
  Complex to Real-Imag : ComplexToRealImag  SampleTime=1e-08
  Constant : Constant  Value=single(0)  OutDataTypeStr=single  SampleTime=1e-08
  Constant1 : Constant  Value=complex(0.5, -0.28867512941360474)  OutDataTypeStr=single  SampleTime=1e-08
  Product : Subsystem
      mask Display: disp('NFP\nmul');
  Product1 : Subsystem
      mask Display: disp('NFP\nmul');
  Product2 : Subsystem
      mask Display: disp('NFP\nmul');
  Product3 : Subsystem
      mask Display: disp('NFP\nmul');
  Product_AC_minus_BD : Subsystem
      mask Display: disp('NFP\nadd');
  Product_AD_plus_BC : Subsystem
      mask Display: disp('NFP\nadd');
  Product_C2ReIm_1 : ComplexToRealImag  SampleTime=1e-08
  Product_C2ReIm_2 : ComplexToRealImag  SampleTime=1e-08
  Product_ReIm2Complex : RealImagToComplex  SampleTime=1e-08
  Real-Imag to Complex : RealImagToComplex  ConstantPart=single(0)  SampleTime=1e-08
  abc   to   alpha_beta_0 : Subsystem
  abc   to   alpha_beta_0_out1_2_term2 : Terminator
  alpha_beta_0   to   abc : Subsystem
  delayMatch{,1..3} (4 alike) : Delay  DelayLength=double(24)  InitialCondition=0  SampleTime=1e-08
  mux : Mux  Inputs=3
  t : Demux  Outputs=3
  Out1 : Outport  SampleTime=1e-08
  wires:
  Complex to Real-Imag/1 -> mux/1
  Complex to Real-Imag/2 -> mux/2
  Constant/1 -> mux/3
  Constant1/1 -> Product_C2ReIm_2/1
  mux/1 -> alpha_beta_0   to   abc/1("alpha, beta, 0  ")
  Product_ReIm2Complex/1 -> Complex to Real-Imag/1
  Real-Imag to Complex/1 -> Product_C2ReIm_1/1
  abc   to   alpha_beta_0/1("alpha, beta, 0 ") -> t/1
  alpha_beta_0   to   abc/1("a, b, c") -> Out1/1
  t/1 -> Real-Imag to Complex/1
  t/2 -> Real-Imag to Complex/2
  t/3 -> abc   to   alpha_beta_0_out1_2_term2/1
  Product_C2ReIm_1/1 -> Product1/1(In1), Product/1(In1)
  Product_C2ReIm_1/2 -> Product3/1(In1), Product2/1(In1)
  delayMatch/1 -> Product/2(In2)
  delayMatch1/1 -> Product1/2(In2)
  delayMatch3/1 -> Product3/2(In2)
  delayMatch2/1 -> Product2/2(In2)
  Product_C2ReIm_2/2 -> delayMatch2/1, delayMatch1/1
  Product_C2ReIm_2/1 -> delayMatch3/1, delayMatch/1
  Product/1(Out1) -> Product_AC_minus_BD/1(In1)
  Product1/1(Out1) -> Product_AD_plus_BC/1(In1)
  Product2/1(Out1) -> Product_AC_minus_BD/2(In2)
  Product3/1(Out1) -> Product_AD_plus_BC/2(In2)
  Product_AC_minus_BD/1(Out1) -> Product_ReIm2Complex/1
  Product_AD_plus_BC/1(Out1) -> Product_ReIm2Complex/2
  In1/1 -> abc   to   alpha_beta_0/1("a, b, c")

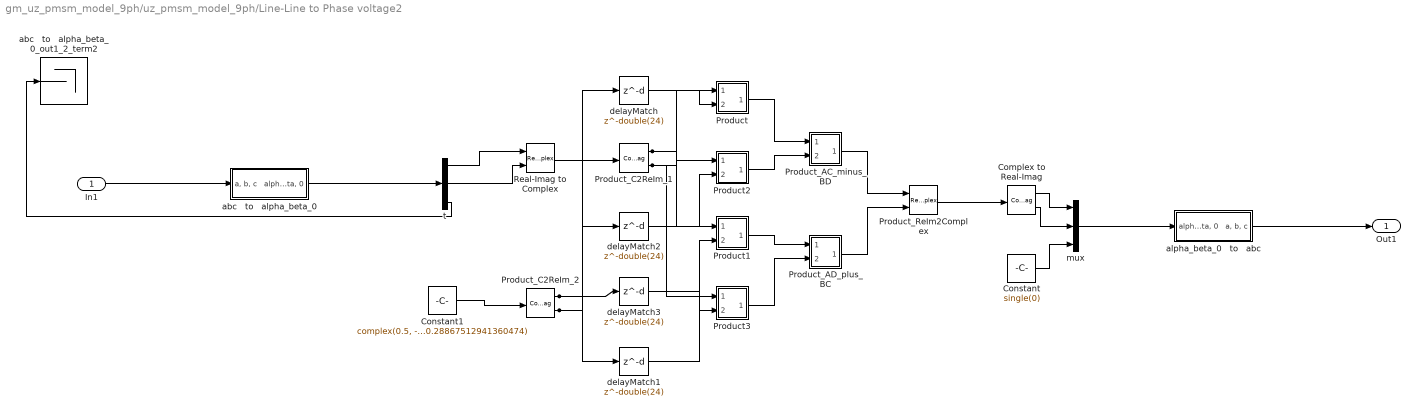
== system gm_uz_pmsm_model_9ph/uz_pmsm_model_9ph/Line-Line to Phase voltage2 ==
  In1 : Inport  OutDataTypeStr=single  PortDimensions=[3]  SampleTime=1e-08
  Complex to Real-Imag : ComplexToRealImag  SampleTime=1e-08
  Constant : Constant  Value=single(0)  OutDataTypeStr=single  SampleTime=1e-08
  Constant1 : Constant  Value=complex(0.5, -0.28867512941360474)  OutDataTypeStr=single  SampleTime=1e-08
  Product : Subsystem
      mask Display: disp('NFP\nmul');
  Product1 : Subsystem
      mask Display: disp('NFP\nmul');
  Product2 : Subsystem
      mask Display: disp('NFP\nmul');
  Product3 : Subsystem
      mask Display: disp('NFP\nmul');
  Product_AC_minus_BD : Subsystem
      mask Display: disp('NFP\nadd');
  Product_AD_plus_BC : Subsystem
      mask Display: disp('NFP\nadd');
  Product_C2ReIm_1 : ComplexToRealImag  SampleTime=1e-08
  Product_C2ReIm_2 : ComplexToRealImag  SampleTime=1e-08
  Product_ReIm2Complex : RealImagToComplex  SampleTime=1e-08
  Real-Imag to Complex : RealImagToComplex  ConstantPart=single(0)  SampleTime=1e-08
  abc   to   alpha_beta_0 : Subsystem
  abc   to   alpha_beta_0_out1_2_term2 : Terminator
  alpha_beta_0   to   abc : Subsystem
  delayMatch{,1..3} (4 alike) : Delay  DelayLength=double(24)  InitialCondition=0  SampleTime=1e-08
  mux : Mux  Inputs=3
  t : Demux  Outputs=3
  Out1 : Outport  SampleTime=1e-08
  wires:
  Complex to Real-Imag/1 -> mux/1
  Complex to Real-Imag/2 -> mux/2
  Constant/1 -> mux/3
  Constant1/1 -> Product_C2ReIm_2/1
  mux/1 -> alpha_beta_0   to   abc/1("alpha, beta, 0  ")
  Product_ReIm2Complex/1 -> Complex to Real-Imag/1
  Real-Imag to Complex/1 -> Product_C2ReIm_1/1
  abc   to   alpha_beta_0/1("alpha, beta, 0 ") -> t/1
  alpha_beta_0   to   abc/1("a, b, c") -> Out1/1
  t/1 -> Real-Imag to Complex/1
  t/2 -> Real-Imag to Complex/2
  t/3 -> abc   to   alpha_beta_0_out1_2_term2/1
  Product_C2ReIm_1/1 -> Product1/1(In1), Product/1(In1)
  Product_C2ReIm_1/2 -> Product3/1(In1), Product2/1(In1)
  delayMatch/1 -> Product/2(In2)
  delayMatch1/1 -> Product1/2(In2)
  delayMatch3/1 -> Product3/2(In2)
  delayMatch2/1 -> Product2/2(In2)
  Product_C2ReIm_2/2 -> delayMatch2/1, delayMatch1/1
  Product_C2ReIm_2/1 -> delayMatch3/1, delayMatch/1
  Product/1(Out1) -> Product_AC_minus_BD/1(In1)
  Product1/1(Out1) -> Product_AD_plus_BC/1(In1)
  Product2/1(Out1) -> Product_AC_minus_BD/2(In2)
  Product3/1(Out1) -> Product_AD_plus_BC/2(In2)
  Product_AC_minus_BD/1(Out1) -> Product_ReIm2Complex/1
  Product_AD_plus_BC/1(Out1) -> Product_ReIm2Complex/2
  In1/1 -> abc   to   alpha_beta_0/1("a, b, c")

== system gm_uz_pmsm_model_9ph/uz_pmsm_model_9ph/Product ==
  In1 : Inport
  In2 : Inport  Port=2
  Product : Product  Inputs=**  OutDataTypeStr=double  SampleTime=1e-08
  Product_pd1 : Delay  DelayLength=6
  Out1 : Outport
  wires:
  In1/1 -> Product/1
  In2/1 -> Product/2
  Product/1 -> Product_pd1/1
  Product_pd1/1 -> Out1/1

== system gm_uz_pmsm_model_9ph/uz_pmsm_model_9ph/Product1 ==
  In1 : Inport
  In2 : Inport  Port=2
  Product1 : Product  Inputs=**  OutDataTypeStr=double  SampleTime=1e-08
  Product1_pd1 : Delay  DelayLength=6
  Out1 : Outport
  wires:
  In1/1 -> Product1/1
  In2/1 -> Product1/2
  Product1/1 -> Product1_pd1/1
  Product1_pd1/1 -> Out1/1

== system gm_uz_pmsm_model_9ph/uz_pmsm_model_9ph/Product10 ==
  In1 : Inport
  In2 : Inport  Port=2
  Product10 : Product  Inputs=**  OutDataTypeStr=double  SampleTime=1e-08
  Product10_pd1 : Delay  DelayLength=6
  Out1 : Outport
  wires:
  In1/1 -> Product10/1
  In2/1 -> Product10/2
  Product10/1 -> Product10_pd1/1
  Product10_pd1/1 -> Out1/1

== system gm_uz_pmsm_model_9ph/uz_pmsm_model_9ph/Product11 ==
  In1 : Inport
  In2 : Inport  Port=2
  Product11 : Product  Inputs=**  OutDataTypeStr=single  SampleTime=1e-08
  Product11_pd1 : Delay  DelayLength=6
  Out1 : Outport
  wires:
  In1/1 -> Product11/1
  In2/1 -> Product11/2
  Product11/1 -> Product11_pd1/1
  Product11_pd1/1 -> Out1/1

== system gm_uz_pmsm_model_9ph/uz_pmsm_model_9ph/Product2 ==
  In1 : Inport
  In2 : Inport  Port=2
  Product2 : Product  Inputs=**  OutDataTypeStr=single  SampleTime=1e-08
  Product2_pd1 : Delay  DelayLength=6
  Out1 : Outport
  wires:
  In1/1 -> Product2/1
  In2/1 -> Product2/2
  Product2/1 -> Product2_pd1/1
  Product2_pd1/1 -> Out1/1

== system gm_uz_pmsm_model_9ph/uz_pmsm_model_9ph/Product3 ==
  In1 : Inport
  In2 : Inport  Port=2
  Product3 : Product  Inputs=**  OutDataTypeStr=single  SampleTime=1e-08
  Product3_pd1 : Delay  DelayLength=6
  Out1 : Outport
  wires:
  In1/1 -> Product3/1
  In2/1 -> Product3/2
  Product3/1 -> Product3_pd1/1
  Product3_pd1/1 -> Out1/1

== system gm_uz_pmsm_model_9ph/uz_pmsm_model_9ph/Product5 ==
  In1 : Inport
  In2 : Inport  Port=2
  Product5 : Product  Inputs=**  OutDataTypeStr=double  SampleTime=1e-08
  Product5_pd1 : Delay  DelayLength=6
  Out1 : Outport
  wires:
  In1/1 -> Product5/1
  In2/1 -> Product5/2
  Product5/1 -> Product5_pd1/1
  Product5_pd1/1 -> Out1/1

== system gm_uz_pmsm_model_9ph/uz_pmsm_model_9ph/Product6 ==
  In1 : Inport
  In2 : Inport  Port=2
  Product6 : Product  Inputs=**  OutDataTypeStr=double  SampleTime=1e-08
  Product6_pd1 : Delay  DelayLength=6
  Out1 : Outport
  wires:
  In1/1 -> Product6/1
  In2/1 -> Product6/2
  Product6/1 -> Product6_pd1/1
  Product6_pd1/1 -> Out1/1

== system gm_uz_pmsm_model_9ph/uz_pmsm_model_9ph/Product7 ==
  In1 : Inport
  In2 : Inport  Port=2
  Product7 : Product  Inputs=**  OutDataTypeStr=double  SampleTime=1e-08
  Product7_pd1 : Delay  DelayLength=6
  Out1 : Outport
  wires:
  In1/1 -> Product7/1
  In2/1 -> Product7/2
  Product7/1 -> Product7_pd1/1
  Product7_pd1/1 -> Out1/1

== system gm_uz_pmsm_model_9ph/uz_pmsm_model_9ph/Product8 ==
  In1 : Inport
  In2 : Inport  Port=2
  Product8 : Product  Inputs=**  OutDataTypeStr=double  SampleTime=1e-08
  Product8_pd1 : Delay  DelayLength=6
  Out1 : Outport
  wires:
  In1/1 -> Product8/1
  In2/1 -> Product8/2
  Product8/1 -> Product8_pd1/1
  Product8_pd1/1 -> Out1/1

== system gm_uz_pmsm_model_9ph/uz_pmsm_model_9ph/Product9 ==
  In1 : Inport
  In2 : Inport  Port=2
  Product9 : Product  Inputs=**  OutDataTypeStr=single  SampleTime=1e-08
  Product9_pd1 : Delay  DelayLength=6
  Out1 : Outport
  wires:
  In1/1 -> Product9/1
  In2/1 -> Product9/2
  Product9/1 -> Product9_pd1/1
  Product9_pd1/1 -> Out1/1

== system gm_uz_pmsm_model_9ph/uz_pmsm_model_9ph/Sine_Cosine ==
  In1 : Inport
  Sine_Cosine : Trigonometry  Operator=sincos  SampleTime=1e-08
  Sine_Cosine_pd1 : Delay  DelayLength=27
  Sine_Cosine_pd2 : Delay  DelayLength=27
  Out1 : Outport
  Out2 : Outport  Port=2
  wires:
  In1/1 -> Sine_Cosine/1
  Sine_Cosine/1 -> Sine_Cosine_pd1/1
  Sine_Cosine_pd1/1 -> Out1/1
  Sine_Cosine/2 -> Sine_Cosine_pd2/1
  Sine_Cosine_pd2/1 -> Out2/1

== system gm_uz_pmsm_model_9ph/uz_pmsm_model_9ph/Sum1 ==
  In1 : Inport
  In2 : Inport  Port=2
  Sum1 : Sum  OutDataTypeStr=single  SampleTime=1e-08
  Sum1_pd1 : Delay  DelayLength=6
  Out1 : Outport
  wires:
  In1/1 -> Sum1/1
  In2/1 -> Sum1/2
  Sum1/1 -> Sum1_pd1/1
  Sum1_pd1/1 -> Out1/1

== system gm_uz_pmsm_model_9ph/uz_pmsm_model_9ph/Sum1_stage2 ==
  In1 : Inport
  In2 : Inport  Port=2
  Sum1_stage2 : Sum  Inputs=+-  OutDataTypeStr=double  SampleTime=1e-08
  Sum1_stage2_pd1 : Delay  DelayLength=6
  Out1 : Outport
  wires:
  In1/1 -> Sum1_stage2/1
  In2/1 -> Sum1_stage2/2
  Sum1_stage2/1 -> Sum1_stage2_pd1/1
  Sum1_stage2_pd1/1 -> Out1/1

== system gm_uz_pmsm_model_9ph/uz_pmsm_model_9ph/Sum1_stage3 ==
  In1 : Inport
  In2 : Inport  Port=2
  Sum1_stage3 : Sum  Inputs=+-  OutDataTypeStr=double  SampleTime=1e-08
  Sum1_stage3_pd1 : Delay  DelayLength=6
  Out1 : Outport
  wires:
  In1/1 -> Sum1_stage3/1
  In2/1 -> Sum1_stage3/2
  Sum1_stage3/1 -> Sum1_stage3_pd1/1
  Sum1_stage3_pd1/1 -> Out1/1

== system gm_uz_pmsm_model_9ph/uz_pmsm_model_9ph/Sum2 ==
  In1 : Inport
  In2 : Inport  Port=2
  Sum2 : Sum  Inputs=+-  OutDataTypeStr=double  SampleTime=1e-08
  Sum2_pd1 : Delay  DelayLength=6
  Out1 : Outport
  wires:
  In1/1 -> Sum2/1
  In2/1 -> Sum2/2
  Sum2/1 -> Sum2_pd1/1
  Sum2_pd1/1 -> Out1/1

== system gm_uz_pmsm_model_9ph/uz_pmsm_model_9ph/Sum3 ==
  In1 : Inport
  In2 : Inport  Port=2
  Sum3 : Sum  OutDataTypeStr=double  SampleTime=1e-08
  Sum3_pd1 : Delay  DelayLength=6
  Out1 : Outport
  wires:
  In1/1 -> Sum3/1
  In2/1 -> Sum3/2
  Sum3/1 -> Sum3_pd1/1
  Sum3_pd1/1 -> Out1/1

== system gm_uz_pmsm_model_9ph/uz_pmsm_model_9ph/Sum31 ==
  In1 : Inport
  In2 : Inport  Port=2
  Sum31 : Sum  OutDataTypeStr=double  SampleTime=1e-08
  Sum31_pd1 : Delay  DelayLength=6
  Out1 : Outport
  wires:
  In1/1 -> Sum31/1
  In2/1 -> Sum31/2
  Sum31/1 -> Sum31_pd1/1
  Sum31_pd1/1 -> Out1/1

== system gm_uz_pmsm_model_9ph/uz_pmsm_model_9ph/Sum310 ==
  In1 : Inport
  In2 : Inport  Port=2
  Sum310 : Sum  OutDataTypeStr=double  SampleTime=1e-08
  Sum310_pd1 : Delay  DelayLength=6
  Out1 : Outport
  wires:
  In1/1 -> Sum310/1
  In2/1 -> Sum310/2
  Sum310/1 -> Sum310_pd1/1
  Sum310_pd1/1 -> Out1/1

== system gm_uz_pmsm_model_9ph/uz_pmsm_model_9ph/Sum32 ==
  In1 : Inport
  In2 : Inport  Port=2
  Sum32 : Sum  OutDataTypeStr=double  SampleTime=1e-08
  Sum32_pd1 : Delay  DelayLength=6
  Out1 : Outport
  wires:
  In1/1 -> Sum32/1
  In2/1 -> Sum32/2
  Sum32/1 -> Sum32_pd1/1
  Sum32_pd1/1 -> Out1/1

== system gm_uz_pmsm_model_9ph/uz_pmsm_model_9ph/Sum33 ==
  In1 : Inport
  In2 : Inport  Port=2
  Sum33 : Sum  Inputs=+-  OutDataTypeStr=single  SampleTime=1e-08
  Sum33_pd1 : Delay  DelayLength=6
  Out1 : Outport
  wires:
  In1/1 -> Sum33/1
  In2/1 -> Sum33/2
  Sum33/1 -> Sum33_pd1/1
  Sum33_pd1/1 -> Out1/1

== system gm_uz_pmsm_model_9ph/uz_pmsm_model_9ph/Sum34 ==
  In1 : Inport
  In2 : Inport  Port=2
  Sum34 : Sum  OutDataTypeStr=double  SampleTime=1e-08
  Sum34_pd1 : Delay  DelayLength=6
  Out1 : Outport
  wires:
  In1/1 -> Sum34/1
  In2/1 -> Sum34/2
  Sum34/1 -> Sum34_pd1/1
  Sum34_pd1/1 -> Out1/1

== system gm_uz_pmsm_model_9ph/uz_pmsm_model_9ph/Sum35 ==
  In1 : Inport
  In2 : Inport  Port=2
  Sum35 : Sum  OutDataTypeStr=double  SampleTime=1e-08
  Sum35_pd1 : Delay  DelayLength=6
  Out1 : Outport
  wires:
  In1/1 -> Sum35/1
  In2/1 -> Sum35/2
  Sum35/1 -> Sum35_pd1/1
  Sum35_pd1/1 -> Out1/1

== system gm_uz_pmsm_model_9ph/uz_pmsm_model_9ph/Sum36 ==
  In1 : Inport
  In2 : Inport  Port=2
  Sum36 : Sum  OutDataTypeStr=double  SampleTime=1e-08
  Sum36_pd1 : Delay  DelayLength=6
  Out1 : Outport
  wires:
  In1/1 -> Sum36/1
  In2/1 -> Sum36/2
  Sum36/1 -> Sum36_pd1/1
  Sum36_pd1/1 -> Out1/1

== system gm_uz_pmsm_model_9ph/uz_pmsm_model_9ph/Sum37 ==
  In1 : Inport
  In2 : Inport  Port=2
  Sum37 : Sum  OutDataTypeStr=double  SampleTime=1e-08
  Sum37_pd1 : Delay  DelayLength=6
  Out1 : Outport
  wires:
  In1/1 -> Sum37/1
  In2/1 -> Sum37/2
  Sum37/1 -> Sum37_pd1/1
  Sum37_pd1/1 -> Out1/1

== system gm_uz_pmsm_model_9ph/uz_pmsm_model_9ph/Sum38 ==
  In1 : Inport
  In2 : Inport  Port=2
  Sum38 : Sum  OutDataTypeStr=double  SampleTime=1e-08
  Sum38_pd1 : Delay  DelayLength=6
  Out1 : Outport
  wires:
  In1/1 -> Sum38/1
  In2/1 -> Sum38/2
  Sum38/1 -> Sum38_pd1/1
  Sum38_pd1/1 -> Out1/1

== system gm_uz_pmsm_model_9ph/uz_pmsm_model_9ph/Sum39 ==
  In1 : Inport
  In2 : Inport  Port=2
  Sum39 : Sum  OutDataTypeStr=double  SampleTime=1e-08
  Sum39_pd1 : Delay  DelayLength=6
  Out1 : Outport
  wires:
  In1/1 -> Sum39/1
  In2/1 -> Sum39/2
  Sum39/1 -> Sum39_pd1/1
  Sum39_pd1/1 -> Out1/1

== system gm_uz_pmsm_model_9ph/uz_pmsm_model_9ph/Sum_stage2 ==
  In1 : Inport
  In2 : Inport  Port=2
  Sum_stage2 : Sum  Inputs=+-  OutDataTypeStr=double  SampleTime=1e-08
  Sum_stage2_pd1 : Delay  DelayLength=6
  Out1 : Outport
  wires:
  In1/1 -> Sum_stage2/1
  In2/1 -> Sum_stage2/2
  Sum_stage2/1 -> Sum_stage2_pd1/1
  Sum_stage2_pd1/1 -> Out1/1

== system gm_uz_pmsm_model_9ph/uz_pmsm_model_9ph/Sum_stage3 ==
  In1 : Inport
  In2 : Inport  Port=2
  Sum_stage3 : Sum  OutDataTypeStr=double  SampleTime=1e-08
  Sum_stage3_pd1 : Delay  DelayLength=6
  Out1 : Outport
  wires:
  In1/1 -> Sum_stage3/1
  In2/1 -> Sum_stage3/2
  Sum_stage3/1 -> Sum_stage3_pd1/1
  Sum_stage3_pd1/1 -> Out1/1
